simulink model "simul"  (R2019a)
settings: Solver=VariableStepAuto  StartTime=0.0  StopTime=10.0  RelTol=1e-3
values from neighbouring files (symbols this model uses):
  Kd = (2*zetac*wc-2*zetam*wm+Rc)/(km*wm^2)    [PIDparameter.m]
  Ki = (Rc.*wc.^2)/(km.*wm^2)    [PIDparameter.m]
  km = 1.115e05/wm^2/120    [PIDparameter.m]    (also in polttt.m = 5.342e05/Wm^2)
  Kp = (wc.^2-wm^2+2*zetac.*wc.*Rc)/(km.*wm^2)    [PIDparameter.m]
  wm = sqrt(1046)    [PIDparameter.m]
  zetam = 34.53/wm/2    [PIDparameter.m]    (also in polttt.m = 250.8/Wm/2)
settings Model: Creator=xde12  LastModifiedBy=xde12

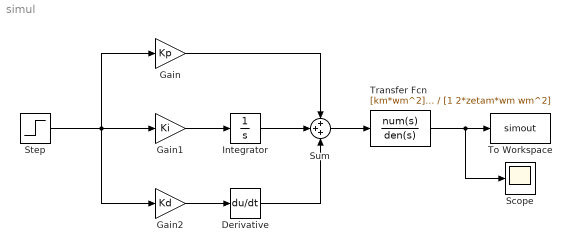
== system simul ==
  Derivative : Derivative
  Gain : Gain  Gain=Kp
  Gain1 : Gain  Gain=Ki
  Gain2 : Gain  Gain=Kd
  Integrator : Integrator
  Scope : Scope
  Step : Step  SampleTime=0
  Sum : Sum  Inputs=+++
  To Workspace : ToWorkspace  VariableName=simout  SaveFormat=Structure With Time  SampleTime=-1
  Transfer Fcn : TransferFcn  Numerator=[km*wm^2]  Denominator=[1 2*zetam*wm wm^2]
  wires:
  Step/1 -> Gain/1, Gain2/1, Gain1/1
  Gain1/1 -> Integrator/1
  Integrator/1 -> Sum/2
  Gain/1 -> Sum/1
  Gain2/1 -> Derivative/1
  Derivative/1 -> Sum/3
  Sum/1 -> Transfer Fcn/1
  Transfer Fcn/1 -> Scope/1, To Workspace/1
